simulink model ""  (R2025b)
settings: Solver=ode4  StartTime=0.0  StopTime=300  FixedStep=0.1  RelTol=1e-3
InitFcn:
  | initialization_2d
values from neighbouring files (symbols this model uses):
  d2r = 0.0174532925199    [DDPG_HybridFlocking_agents8-4-1.mat]    (also in flocking_learning.m; initialization_2d.m)
  g = spec(2)    [ActualOutput.m]    (also in DDPG_HybridFlocking_agents8-4-1.mat = 9.806; ModelSwarm.m; initialization.m = 9.806; initialization_2d.m = 9.806)
  m = spec(1)    [ActualOutput.m]    (also in DDPG_HybridFlocking_agents8-4-1.mat = 5; ModelSwarm.m; initialization.m = 15; initialization_2d.m = 5)
  state0 = [435.012620465 721.15936685 20 2.59881408791 0 187.945467124 786.05177403 20 2.90689824266 0 842.493878094 376.880931214 ... (25 elements, 5x5)]    [DDPG_HybridFlocking_agents8-4-1.mat]    (also in flocking_learning.m = zeros(5, N); initialization.m = [x0; y0; z0; V0; gam0; psi0]; initialization_2d.m = [x0; y0; V0; psi0; bank0])
libraries: simulink_extras x10, rllib x6
(part 1 of 2)
settings Model: Creator=chang  LastModifiedBy=laaa

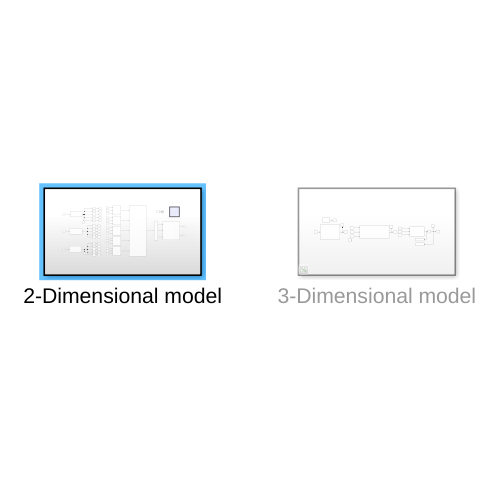
[thumbnail: Simulink's stored preview of the top-level diagram]
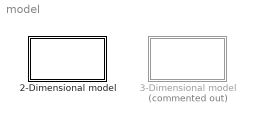
== system model ==
  2-Dimensional model : Subsystem
  3-Dimensional model : Subsystem  Commented=on

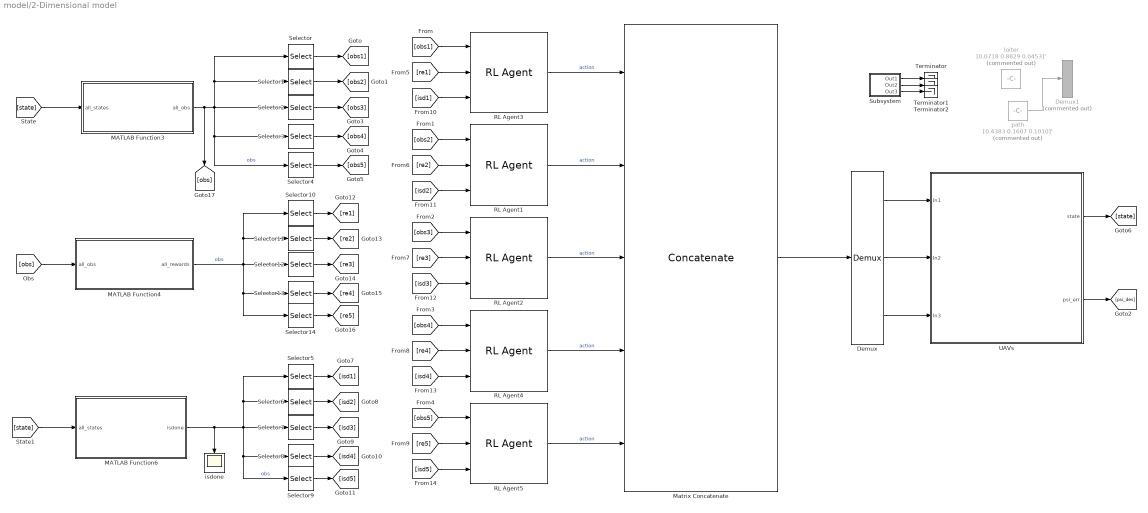
== system model/2-Dimensional model ==
  Demux : Demux  Outputs=3
  Demux1 : Demux  Commented=on  Outputs=3
  MATLAB Function3 : MATLAB Function  TreatAsAtomicUnit=on
  MATLAB Function4 : MATLAB Function  TreatAsAtomicUnit=on
  MATLAB Function6 : MATLAB Function  TreatAsAtomicUnit=on
  Matrix Concatenate : Concatenate  NumInputs=5  Mode=Multidimensional array  ConcatenateDimension=2
  RL Agent{1..5} (5 alike) : rllib/RL Agent  Agent=agent  ExternalActionAsInput=off  ProvideLastAction=off  ProvideCumRwd=off  TreatAsDirectFeedthrough=on  UseStrictObservationDataTypes=off
  Selector : Selector  NumberOfDimensions=2  InputPortWidth=3  IndexOptions=Index vector (dialog),Index vector (dialog)  Indices=1:6,1  OutputSizes=1,1
  Selector1 : Selector  NumberOfDimensions=2  InputPortWidth=3  IndexOptions=Index vector (dialog),Index vector (dialog)  Indices=1:6,2  OutputSizes=1,1
  Selector10 : Selector  NumberOfDimensions=2  InputPortWidth=3  IndexOptions=Index vector (dialog),Index vector (dialog)  Indices=1,1  OutputSizes=1,1
  Selector11 : Selector  NumberOfDimensions=2  InputPortWidth=3  IndexOptions=Index vector (dialog),Index vector (dialog)  Indices=1,2  OutputSizes=1,1
  Selector12 : Selector  NumberOfDimensions=2  InputPortWidth=3  IndexOptions=Index vector (dialog),Index vector (dialog)  Indices=1,3  OutputSizes=1,1
  Selector13 : Selector  NumberOfDimensions=2  InputPortWidth=3  IndexOptions=Index vector (dialog),Index vector (dialog)  Indices=1,4  OutputSizes=1,1
  Selector14 : Selector  NumberOfDimensions=2  InputPortWidth=3  IndexOptions=Index vector (dialog),Index vector (dialog)  Indices=1,5  OutputSizes=1,1
  Selector2 : Selector  NumberOfDimensions=2  InputPortWidth=3  IndexOptions=Index vector (dialog),Index vector (dialog)  Indices=1:6,3  OutputSizes=1,1
  Selector3 : Selector  NumberOfDimensions=2  InputPortWidth=3  IndexOptions=Index vector (dialog),Index vector (dialog)  Indices=1:6,4  OutputSizes=1,1
  Selector4 : Selector  NumberOfDimensions=2  InputPortWidth=3  IndexOptions=Index vector (dialog),Index vector (dialog)  Indices=1:6,5  OutputSizes=1,1
  Selector5 : Selector  NumberOfDimensions=2  InputPortWidth=3  IndexOptions=Index vector (dialog),Index vector (dialog)  Indices=1,1  OutputSizes=1,1
  Selector6 : Selector  NumberOfDimensions=2  InputPortWidth=3  IndexOptions=Index vector (dialog),Index vector (dialog)  Indices=1,2  OutputSizes=1,1
  Selector7 : Selector  NumberOfDimensions=2  InputPortWidth=3  IndexOptions=Index vector (dialog),Index vector (dialog)  Indices=1,3  OutputSizes=1,1
  Selector8 : Selector  NumberOfDimensions=2  InputPortWidth=3  IndexOptions=Index vector (dialog),Index vector (dialog)  Indices=1,4  OutputSizes=1,1
  Selector9 : Selector  NumberOfDimensions=2  InputPortWidth=3  IndexOptions=Index vector (dialog),Index vector (dialog)  Indices=1,5  OutputSizes=1,1
  Subsystem : Subsystem
  Terminator : Terminator
  Terminator1 : Terminator
  Terminator2 : Terminator
  UAVs : Subsystem
  isdone : Scope
      settings: TimeSpan=300  ActiveDisplayYMinimum=-1  ActiveDisplayYMaximum=1  DataLoggingVariableName=ScopeData23
  loiter : Constant  Commented=on  Value=[0.0718 0.8829 0.0453]'
  path : Constant  Commented=on  Value=[0.4383 0.1607 0.1010]'
  wires:
  Demux/3 -> UAVs/3(In3)
  [state] -> MATLAB Function3/1(all_states)
  Demux/2 -> UAVs/2(In2)
  UAVs/2(psi_err) -> [psi_des]
  [obs] -> MATLAB Function4/1(all_obs)
  UAVs/1(state) -> [state]
  path/1 -> Demux1/1
  Demux/1 -> UAVs/1(In1)
  MATLAB Function3/1(all_obs) -> Selector2/1, Selector3/1, Selector4/1, Selector/1, Selector1/1, [obs]  "obs"
  Subsystem/1(Out1) -> Terminator/1
  Subsystem/2(Out2) -> Terminator1/1
  Subsystem/3(Out3) -> Terminator2/1
  [state] -> MATLAB Function6/1(all_states)
  MATLAB Function4/1(all_rewards) -> Selector10/1, Selector11/1, Selector12/1, Selector13/1, Selector14/1  "obs"
  Selector1/1 -> [obs2]
  Selector/1 -> [obs1]
  Selector2/1 -> [obs3]
  Selector3/1 -> [obs4]
  Selector14/1 -> [re5]
  Selector13/1 -> [re4]
  Selector12/1 -> [re3]
  Selector11/1 -> [re2]
  Selector10/1 -> [re1]
  Selector4/1 -> [obs5]
  Selector5/1 -> [isd1]
  Selector9/1 -> [isd5]
  Selector8/1 -> [isd4]
  MATLAB Function6/1(isdone) -> Selector5/1, Selector6/1, Selector7/1, Selector8/1, Selector9/1, isdone/1  "obs"
  Selector6/1 -> [isd2]
  Selector7/1 -> [isd3]
  [re1] -> RL Agent3/2
  [isd1] -> RL Agent3/3
  [obs1] -> RL Agent3/1
  [obs2] -> RL Agent1/1
  [re2] -> RL Agent1/2
  [isd2] -> RL Agent1/3
  [obs3] -> RL Agent2/1
  [re3] -> RL Agent2/2
  [isd3] -> RL Agent2/3
  [obs4] -> RL Agent4/1
  [re4] -> RL Agent4/2
  [isd4] -> RL Agent4/3
  [obs5] -> RL Agent5/1
  [re5] -> RL Agent5/2
  [isd5] -> RL Agent5/3
  RL Agent2/1 -> Matrix Concatenate/3  "action"
  RL Agent4/1 -> Matrix Concatenate/4  "action"
  RL Agent1/1 -> Matrix Concatenate/2  "action"
  RL Agent5/1 -> Matrix Concatenate/5  "action"
  RL Agent3/1 -> Matrix Concatenate/1  "action"
  Matrix Concatenate/1 -> Demux/1

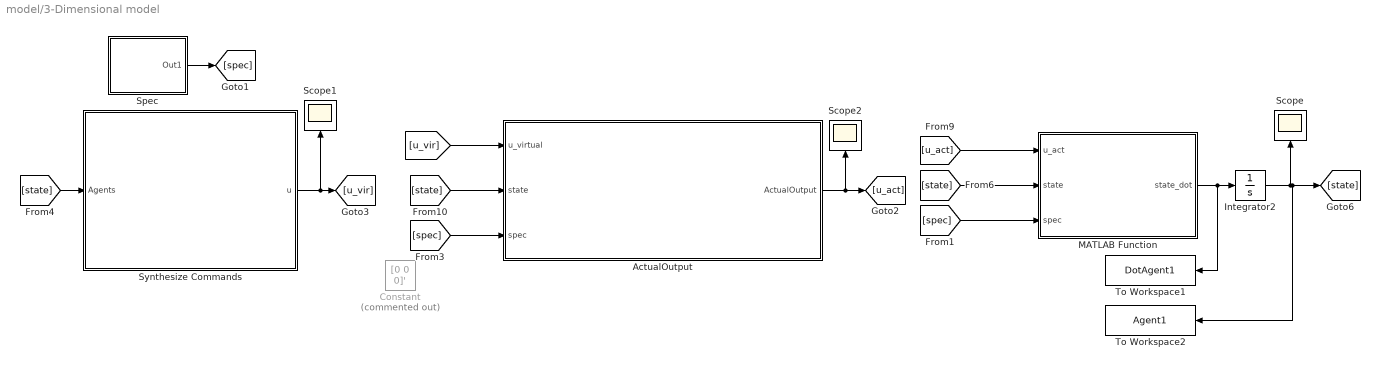
== system model/3-Dimensional model ==
  ActualOutput : Subsystem
  Constant : Constant  Commented=on  Value=[0 0 0]'
  Integrator2 : Integrator  InitialCondition=state0  UpperSaturationLimit=[10^6 ;10^6 ;10^6 ;30 ;15 ;10^6]  LowerSaturationLimit=[-10^6; -10^6 ;-10^6; 0; -15 ;-10^6]'
  MATLAB Function : MATLAB Function  TreatAsAtomicUnit=on
  Scope : Scope
      settings: ActiveDisplayYMinimum=-1796.4442274835574  ActiveDisplayYMaximum=1827.1129411617226
  Scope1 : Scope
      settings: ActiveDisplayYMinimum=-0.625  ActiveDisplayYMaximum=0.625
  Scope2 : Scope
      settings: ActiveDisplayYMinimum=-543.50698903671855  ActiveDisplayYMaximum=2400.6247544411835  DataLoggingVariableName=ScopeData2
  Spec : Subsystem
  Synthesize Commands : Subsystem
  To Workspace1 : ToWorkspace  VariableName=DotAgent1  SaveFormat=Timeseries  SampleTime=-1
  To Workspace2 : ToWorkspace  VariableName=Agent1  SaveFormat=Timeseries  SampleTime=-1
  wires:
  [spec] -> MATLAB Function/3(spec)
  Synthesize Commands/1(u) -> Scope1/1, [u_vir]
  [state] -> ActualOutput/2(state)
  [spec] -> ActualOutput/3(spec)
  [state] -> Synthesize Commands/1(Agents)
  Integrator2/1 -> [state], To Workspace2/1, Scope/1
  [u_vir] -> ActualOutput/1(u_virtual)
  ActualOutput/1(ActualOutput) -> Scope2/1, [u_act]
  MATLAB Function/1(state_dot) -> To Workspace1/1, Integrator2/1
  Spec/1(Out1) -> [spec]
  [state] -> MATLAB Function/2(state)
  [u_act] -> MATLAB Function/1(u_act)

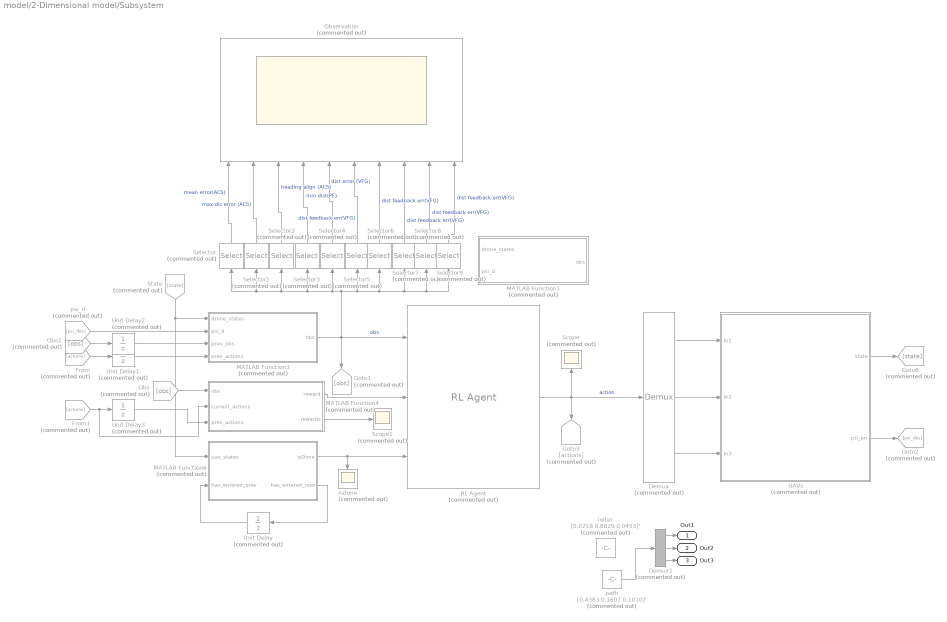
== system model/2-Dimensional model/Subsystem ==
  Demux : Demux  Commented=on  Outputs=3
  Demux1 : Demux  Commented=on  Outputs=3
  From : From  Commented=on  GotoTag=actions
  From1 : From  Commented=on  GotoTag=actions
  Goto1 : Goto  Commented=on  GotoTag=obs
  Goto2 : Goto  Commented=on  GotoTag=psi_des
  Goto3 : Goto  Commented=on  GotoTag=actions
  Goto6 : Goto  Commented=on  GotoTag=state
  MATLAB Function1 : MATLAB Function  Commented=on  TreatAsAtomicUnit=on
  MATLAB Function3 : MATLAB Function  Commented=on  TreatAsAtomicUnit=on
  MATLAB Function4 : MATLAB Function  Commented=on  TreatAsAtomicUnit=on
  MATLAB Function6 : MATLAB Function  Commented=on  TreatAsAtomicUnit=on
  Obs : From  Commented=on  GotoTag=obs
  Obs1 : From  Commented=on  GotoTag=obs
  Observation : Scope  Commented=on  NumInputPorts=10
      settings: TimeSpan=300  TimeDisplayOffset=1  ActiveDisplayYMinimum=0.24464995382973423  ActiveDisplayYMaximum=1.0839277829078073  DataLoggingVariableName=ScopeData20
  RL Agent : rllib/RL Agent  Commented=on  Agent=agent  ExternalActionAsInput=off  ProvideLastAction=off  ProvideCumRwd=off  TreatAsDirectFeedthrough=on  UseStrictObservationDataTypes=off
  Scope : Scope  Commented=on
      settings: TimeSpan=300  ActiveDisplayYMinimum=0.99966044723987579  ActiveDisplayYMaximum=1.0000375956296921  DataLoggingVariableName=ScopeData15
  Scope1 : Scope  Commented=on
      settings: TimeSpan=300  ActiveDisplayYMinimum=-10.882528944657471  ActiveDisplayYMaximum=4.416291277713289  DataLoggingVariableName=ScopeData17
  Selector : Selector  Commented=on  NumberOfDimensions=2  InputPortWidth=3  IndexOptions=Index vector (dialog),Index vector (dialog)  Indices=1,1  OutputSizes=1,1
  Selector1 : Selector  Commented=on  NumberOfDimensions=2  InputPortWidth=3  IndexOptions=Index vector (dialog),Index vector (dialog)  Indices=2,1  OutputSizes=1,1
  Selector2 : Selector  Commented=on  NumberOfDimensions=2  InputPortWidth=3  IndexOptions=Index vector (dialog),Index vector (dialog)  Indices=3,1  OutputSizes=1,1
  Selector3 : Selector  Commented=on  NumberOfDimensions=2  InputPortWidth=3  IndexOptions=Index vector (dialog),Index vector (dialog)  Indices=4,1  OutputSizes=1,1
  Selector4 : Selector  Commented=on  NumberOfDimensions=2  InputPortWidth=3  IndexOptions=Index vector (dialog),Index vector (dialog)  Indices=5,1  OutputSizes=1,1
  Selector5 : Selector  Commented=on  NumberOfDimensions=2  InputPortWidth=3  IndexOptions=Index vector (dialog),Index vector (dialog)  Indices=6,1  OutputSizes=1,1
  Selector6 : Selector  Commented=on  NumberOfDimensions=2  InputPortWidth=3  IndexOptions=Index vector (dialog),Index vector (dialog)  Indices=7,1  OutputSizes=1,1
  Selector7 : Selector  Commented=on  NumberOfDimensions=2  InputPortWidth=3  IndexOptions=Index vector (dialog),Index vector (dialog)  Indices=8,1  OutputSizes=1,1
  Selector8 : Selector  Commented=on  NumberOfDimensions=2  InputPortWidth=3  IndexOptions=Index vector (dialog),Index vector (dialog)  Indices=9,1  OutputSizes=1,1
  Selector9 : Selector  Commented=on  NumberOfDimensions=2  InputPortWidth=3  IndexOptions=Index vector (dialog),Index vector (dialog)  Indices=10,1  OutputSizes=1,1
  State : From  Commented=on  GotoTag=state
  UAVs : Subsystem  Commented=on
  Unit Delay{,1..3} (4 alike) : UnitDelay  Commented=on  SampleTime=-1  HasFrameUpgradeWarning=on
  isdone : Scope  Commented=on
      settings: TimeSpan=300  ActiveDisplayYMinimum=-1  ActiveDisplayYMaximum=1  DataLoggingVariableName=ScopeData12
  loiter : Constant  Commented=on  Value=[0.0718 0.8829 0.0453]'
  path : Constant  Commented=on  Value=[0.4383 0.1607 0.1010]'
  psi_d : From  Commented=on  GotoTag=psi_des
  Out1 : Outport
  Out2 : Outport  Port=2
  Out3 : Outport  Port=3
  wires:
  Unit Delay1/1 -> MATLAB Function3/4(prev_actions)
  Demux/3 -> UAVs/3(In3)
  Obs1/1 -> Unit Delay2/1
  MATLAB Function4/1(reward) -> RL Agent/2
  Selector/1 -> Observation/1  "mean error(ACS)"
  Demux/1 -> UAVs/1(In1)
  From1/1 -> MATLAB Function4/2(current_actions), Unit Delay3/1
  Selector6/1 -> Observation/7  "dist feedback err(VFG)"
  MATLAB Function6/2(has_entered_now) -> Unit Delay/1
  Selector2/1 -> Observation/3  "heading align (ACS)"
  State/1 -> MATLAB Function6/1(uav_states), MATLAB Function3/1(drone_states)
  Selector9/1 -> Observation/10  "dist feedback err(VFG)"
  RL Agent/1 -> Goto3/1, Scope/1, Demux/1  "action"
  Selector1/1 -> Observation/2  "max dis error (ACS)"
  MATLAB Function6/1(isDone) -> RL Agent/3, isdone/1
  From/1 -> Unit Delay1/1
  UAVs/1(state) -> Goto6/1
  Unit Delay2/1 -> MATLAB Function3/3(prev_obs)
  Selector7/1 -> Observation/8  "dist feedback err(VFG)"
  Demux1/2 -> Out2/1
  path/1 -> Demux1/1
  Selector3/1 -> Observation/4  "min dist(PF)"
  MATLAB Function3/1(obs) -> RL Agent/1, Goto1/1, Selector9/1, Selector8/1, Selector7/1, Selector6/1, Selector5/1, Selector/1, Selector1/1, Selector2/1, Selector3/1, Selector4/1  "obs"
  Demux1/1 -> Out1/1
  Demux/2 -> UAVs/2(In2)
  MATLAB Function4/2(rewards) -> Scope1/1
  psi_d/1 -> MATLAB Function3/2(psi_d)
  Unit Delay3/1 -> MATLAB Function4/3(prev_actions)
  UAVs/2(psi_err) -> Goto2/1
  Demux1/3 -> Out3/1
  Unit Delay/1 -> MATLAB Function6/2(has_entered_prev)
  Selector5/1 -> Observation/6  "dist feedback err(VFG)"
  Selector8/1 -> Observation/9  "dist feedback err(VFG)"
  Obs/1 -> MATLAB Function4/1(obs)
  Selector4/1 -> Observation/5  "dist error (VFG)"

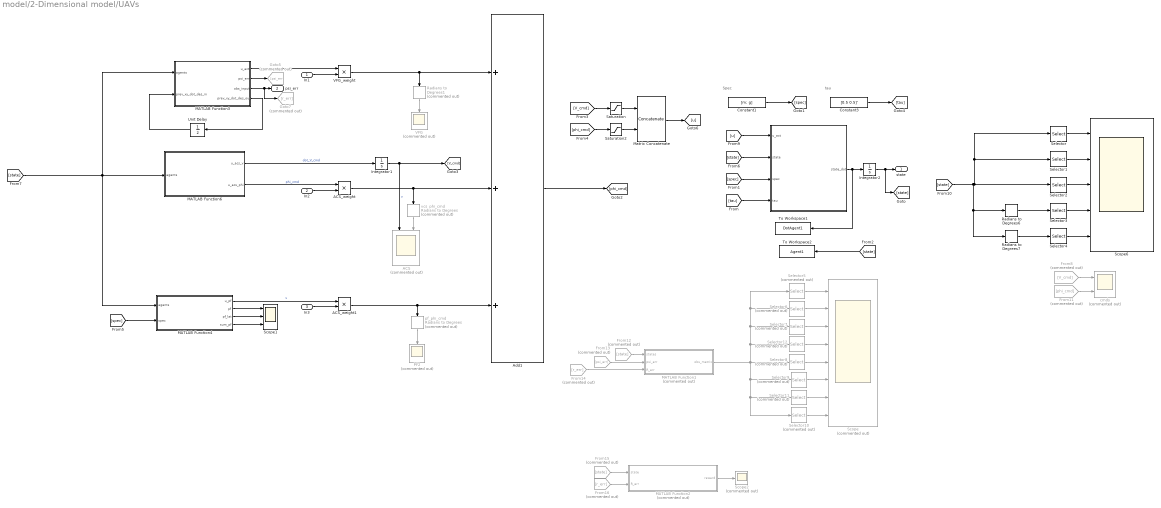
== system model/2-Dimensional model/UAVs ==
  note: Spec
  note: tau
  In1 : Inport
  In2 : Inport  Port=2
  In3 : Inport  Port=3
  " " : MATLAB Function  TreatAsAtomicUnit=on
  ACS : Scope  Commented=on  NumInputPorts=2
      settings: ActiveDisplayYMinimum=-23.869601726691815  ActiveDisplayYMaximum=64.370407175335345  DataLoggingVariableName=ScopeData9
  ACS_weight : Product
  ACS_weight1 : Product
  Add1 : Sum  Inputs=+++
  Constant1 : Constant  Value=[m; g]
  Constant3 : Constant  Value=[0.5 0.5]'
  From11 : From  Commented=on  GotoTag=phi_cmd
  From12 : From  Commented=on  GotoTag=state
  From13 : From  Commented=on  GotoTag=psi_err
  From14 : From  Commented=on  GotoTag=r_err
  From15 : From  Commented=on  GotoTag=state
  From16 : From  Commented=on  GotoTag=r_err
  From8 : From  Commented=on  GotoTag=V_cmd
  Goto5 : Goto  Commented=on  GotoTag=psi_err
  Goto7 : Goto  Commented=on  GotoTag=r_err
  Integrator1 : Integrator  LimitOutput=on  UpperSaturationLimit=35*ones(1,10)  LowerSaturationLimit=15*ones(1,10)
  Integrator2 : Integrator  InitialCondition=state0  LimitOutput=on  UpperSaturationLimit=[10^6; 10^6; 35; 10^6; 30*d2r ]*ones(1,10)  LowerSaturationLimit=[-10^6; -10^6; 15; -10^6; -30*d2r ]*ones(1,10)
  MATLAB Function1 : MATLAB Function  Commented=on  TreatAsAtomicUnit=on
  MATLAB Function2 : MATLAB Function  Commented=on  TreatAsAtomicUnit=on
  MATLAB Function3 : MATLAB Function  TreatAsAtomicUnit=on
  MATLAB Function4 : MATLAB Function  TreatAsAtomicUnit=on
  MATLAB Function6 : MATLAB Function  TreatAsAtomicUnit=on
  Matrix Concatenate : Concatenate  Mode=Multidimensional array
  PF2 : Scope  Commented=on
      settings: TimeSpan=300  ActiveDisplayYMinimum=-44.741397355611163  ActiveDisplayYMaximum=44.744942341518566  DataLoggingVariableName=ScopeData10
  Radians to Degrees1 : simulink_extras/Transformations/Radians to Degrees  Commented=on
  Radians to Degrees6 : simulink_extras/Transformations/Radians to Degrees
  Radians to Degrees7 : simulink_extras/Transformations/Radians to Degrees
  Saturation : Saturate  UpperLimit=35*ones(1,10)  LowerLimit=15*ones(1,10)
  Saturation2 : Saturate  UpperLimit=30*d2r*ones(1,10)  LowerLimit=-30*d2r*ones(1,10)  LinearizeAsGain=off
  Scope : Scope  Commented=on  NumInputPorts=8
      settings: ActiveDisplayString=4  ActiveDisplayYMinimum=0.29571525373676022  ActiveDisplayYMaximum=1.0782538606959156  DataLoggingVariableName=ScopeData18
  Scope1 : Scope  NumInputPorts=3
      settings: ActiveDisplayYMinimum=-1  ActiveDisplayYMaximum=1  DataLoggingVariableName=ScopeData16
  Scope2 : Scope  Commented=on
      settings: ActiveDisplayYMinimum=-109.38583360755611  ActiveDisplayYMaximum=7.8590338705691378  DataLoggingVariableName=ScopeData19
  Scope6 : Scope  NumInputPorts=5
      settings: TimeSpan=300  ActiveDisplayString=5  ShowGrid=off  ActiveDisplayYMinimum=-37.354494394302066  ActiveDisplayYMaximum=37.435243344907619  YLabel=Bank angle (deg)  DataLoggingVariableName=ScopeData13
  Selector : Selector  NumberOfDimensions=2  InputPortWidth=3  IndexOptions=Index vector (dialog),Index vector (dialog)  Indices=1,1:10  OutputSizes=1,1
  Selector1 : Selector  NumberOfDimensions=2  InputPortWidth=3  IndexOptions=Index vector (dialog),Index vector (dialog)  Indices=2,1:10  OutputSizes=1,1
  Selector10 : Selector  Commented=on  NumberOfDimensions=2  InputPortWidth=3  IndexOptions=Index vector (dialog),Index vector (dialog)  Indices=8,1:5  OutputSizes=1,1
  Selector11 : Selector  Commented=on  NumberOfDimensions=2  InputPortWidth=3  IndexOptions=Index vector (dialog),Index vector (dialog)  Indices=7,1:5  OutputSizes=1,1
  Selector12 : Selector  Commented=on  NumberOfDimensions=2  InputPortWidth=3  IndexOptions=Index vector (dialog),Index vector (dialog)  Indices=4,1:5  OutputSizes=1,1
  Selector2 : Selector  NumberOfDimensions=2  InputPortWidth=3  IndexOptions=Index vector (dialog),Index vector (dialog)  Indices=3,1:10  OutputSizes=1,1
  Selector3 : Selector  NumberOfDimensions=2  InputPortWidth=3  IndexOptions=Index vector (dialog),Index vector (dialog)  Indices=4,1:10  OutputSizes=1,1
  Selector4 : Selector  NumberOfDimensions=2  InputPortWidth=3  IndexOptions=Index vector (dialog),Index vector (dialog)  Indices=5,1:10  OutputSizes=1,1
  Selector5 : Selector  Commented=on  NumberOfDimensions=2  InputPortWidth=3  IndexOptions=Index vector (dialog),Index vector (dialog)  Indices=1,1:5  OutputSizes=1,1
  Selector6 : Selector  Commented=on  NumberOfDimensions=2  InputPortWidth=3  IndexOptions=Index vector (dialog),Index vector (dialog)  Indices=2,1:5  OutputSizes=1,1
  Selector7 : Selector  Commented=on  NumberOfDimensions=2  InputPortWidth=3  IndexOptions=Index vector (dialog),Index vector (dialog)  Indices=3,1:5  OutputSizes=1,1
  Selector8 : Selector  Commented=on  NumberOfDimensions=2  InputPortWidth=3  IndexOptions=Index vector (dialog),Index vector (dialog)  Indices=5,1:5  OutputSizes=1,1
  Selector9 : Selector  Commented=on  NumberOfDimensions=2  InputPortWidth=3  IndexOptions=Index vector (dialog),Index vector (dialog)  Indices=6,1:5  OutputSizes=1,1
  To Workspace1 : ToWorkspace  VariableName=DotAgent1  SaveFormat=Timeseries  SampleTime=-1
  To Workspace2 : ToWorkspace  VariableName=Agent1  SaveFormat=Timeseries  SampleTime=-1
  Unit Delay : UnitDelay  SampleTime=-1  HasFrameUpgradeWarning=on
  VFG : Scope  Commented=on
      settings: ActiveDisplayYMinimum=-2.2311275771009429  ActiveDisplayYMaximum=1.6680942354459041  DataLoggingVariableName=ScopeData8
  VFG_weight : Product
  cmds : Scope  Commented=on  NumInputPorts=2
      settings: ActiveDisplayYMinimum=-0.21104649012249277  ActiveDisplayYMaximum=0.44117626715669322  DataLoggingVariableName=ScopeData14
  pf_phi_cmd : simulink_extras/Transformations/Radians to Degrees  Commented=on
  vcs_phi_cmd : simulink_extras/Transformations/Radians to Degrees  Commented=on
  state : Outport
  psi_err : Outport  Port=2
  wires:
  " "/1(state_dot) -> To Workspace1/1, Integrator2/1
  [state] -> MATLAB Function4/1(agents), MATLAB Function3/1(agents), MATLAB Function6/1(agents)
  [spec] -> MATLAB Function4/2(spec)
  MATLAB Function4/1(u_pf) -> ACS_weight1/1  "v"
  MATLAB Function6/2(u_acs_phi) -> ACS_weight/1  "phi_cmd"
  MATLAB Function3/1(u_act) -> VFG_weight/1
  In1/1 -> VFG_weight/2
  VFG_weight/1 -> Radians to Degrees1/1, Add1/1
  Radians to Degrees1/1 -> VFG/1
  MATLAB Function6/1(u_acs_v) -> Integrator1/1  "dot_V_cmd"
  Integrator1/1 -> ACS/1, [V_cmd]  "v"
  ACS_weight/1 -> Add1/2, vcs_phi_cmd/1
  In2/1 -> ACS_weight/2
  vcs_phi_cmd/1 -> ACS/2
  MATLAB Function4/4(sum_pf) -> Scope1/3
  MATLAB Function4/3(pf_lat) -> Scope1/2
  MATLAB Function4/2(pf) -> Scope1/1
  In3/1 -> ACS_weight1/2
  ACS_weight1/1 -> pf_phi_cmd/1, Add1/3
  pf_phi_cmd/1 -> PF2/1
  Add1/1 -> [phi_cmd]
  [V_cmd] -> Saturation/1
  [phi_cmd] -> Saturation2/1
  Saturation/1 -> Matrix Concatenate/1
  Saturation2/1 -> Matrix Concatenate/2
  Matrix Concatenate/1 -> [u]
  [u] -> " "/1(u_act)
  [state] -> " "/2(state)
  [spec] -> " "/3(spec)
  [tau] -> " "/4(tau)
  Constant1/1 -> [spec]
  Constant3/1 -> [tau]
  Integrator2/1 -> [state], state/1
  [state] -> To Workspace2/1
  Selector/1 -> Scope6/1
  Selector1/1 -> Scope6/2
  Selector2/1 -> Scope6/3
  Selector3/1 -> Scope6/4
  Selector4/1 -> Scope6/5
  [state] -> Selector2/1, Selector/1, Selector1/1, Radians to Degrees6/1, Radians to Degrees7/1
  Radians to Degrees6/1 -> Selector3/1
  Radians to Degrees7/1 -> Selector4/1
  From8/1 -> cmds/1
  From11/1 -> cmds/2
  MATLAB Function3/2(psi_err) -> Goto5/1
  MATLAB Function3/3(obs_input) -> Goto7/1, psi_err/1
  From12/1 -> MATLAB Function1/1(states)
  From13/1 -> MATLAB Function1/2(psi_err)
  From14/1 -> MATLAB Function1/3(R_err)
  MATLAB Function1/1(obs_matrix) -> Selector6/1, Selector5/1, Selector7/1, Selector12/1, Selector8/1, Selector9/1, Selector10/1, Selector11/1
  Selector9/1 -> Scope/6
  Selector11/1 -> Scope/7
  Selector10/1 -> Scope/8
  Selector5/1 -> Scope/1
  Selector6/1 -> Scope/2
  Selector7/1 -> Scope/3
  Selector12/1 -> Scope/4
  Selector8/1 -> Scope/5
  From15/1 -> MATLAB Function2/1(state)
  From16/1 -> MATLAB Function2/2(R_err)
  MATLAB Function2/1(reward) -> Scope2/1
  MATLAB Function3/4(prev_xy_dot_des_out) -> Unit Delay/1
  Unit Delay/1 -> MATLAB Function3/2(prev_xy_dot_des_in)

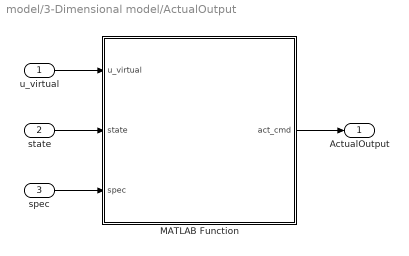
== system model/3-Dimensional model/ActualOutput ==
  u_virtual : Inport
  state : Inport  Port=2
  spec : Inport  Port=3
  MATLAB Function : MATLAB Function  TreatAsAtomicUnit=on
  ActualOutput : Outport
  wires:
  u_virtual/1 -> MATLAB Function/1(u_virtual)
  state/1 -> MATLAB Function/2(state)
  spec/1 -> MATLAB Function/3(spec)
  MATLAB Function/1(act_cmd) -> ActualOutput/1

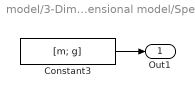
== system model/3-Dimensional model/Spec ==
  Constant3 : Constant  Value=[m; g]
  Out1 : Outport
  wires:
  Constant3/1 -> Out1/1

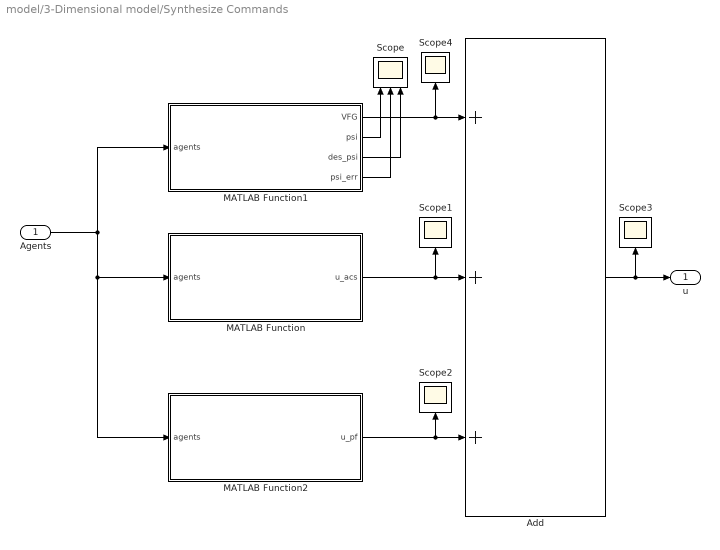
== system model/3-Dimensional model/Synthesize Commands ==
  Agents : Inport
  Add : Sum  Inputs=+++
  MATLAB Function : MATLAB Function  TreatAsAtomicUnit=on
  MATLAB Function1 : MATLAB Function  TreatAsAtomicUnit=on
  MATLAB Function2 : MATLAB Function  TreatAsAtomicUnit=on
  Scope : Scope  NumInputPorts=3
      settings: ActiveDisplayYMinimum=-7.5463075515448264  ActiveDisplayYMaximum=36.500847150660185  DataLoggingVariableName=ScopeData3
  Scope{1..4} (4 alike) : Scope
      Scope1 settings: ActiveDisplayYMinimum=-13.729609129882078  ActiveDisplayYMaximum=15.057455581515576  DataLoggingVariableName=ScopeData4
      Scope2 settings: ActiveDisplayYMinimum=-2.3665763647029392  ActiveDisplayYMaximum=2.4298902475942277  DataLoggingVariableName=ScopeData5
      Scope3 settings: ActiveDisplayYMinimum=-7.2803454393817137  ActiveDisplayYMaximum=5.3802620907689036  DataLoggingVariableName=ScopeData6
      Scope4 settings: ActiveDisplayYMinimum=-15.035450003897875  ActiveDisplayYMaximum=9.9786981173949183  DataLoggingVariableName=ScopeData7
  u : Outport
  wires:
  Agents/1 -> MATLAB Function2/1(agents), MATLAB Function/1(agents), MATLAB Function1/1(agents)
  MATLAB Function1/2(psi) -> Scope/1
  MATLAB Function1/3(des_psi) -> Scope/3
  MATLAB Function1/4(psi_err) -> Scope/2
  MATLAB Function1/1(VFG) -> Add/1, Scope4/1
  MATLAB Function/1(u_acs) -> Scope1/1, Add/2
  MATLAB Function2/1(u_pf) -> Add/3, Scope2/1
  Add/1 -> Scope3/1, u/1

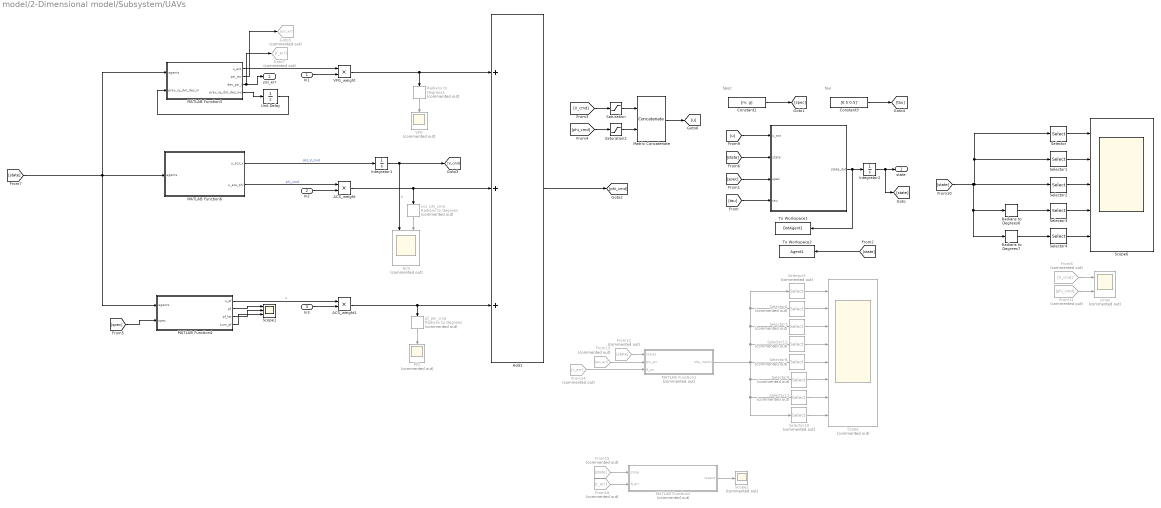
== system model/2-Dimensional model/Subsystem/UAVs ==
  note: Spec
  note: tau
  In1 : Inport
  In2 : Inport  Port=2
  In3 : Inport  Port=3
  " " : MATLAB Function  TreatAsAtomicUnit=on
  ACS : Scope  Commented=on  NumInputPorts=2
      settings: ActiveDisplayYMinimum=-23.869601726691815  ActiveDisplayYMaximum=64.370407175335345  DataLoggingVariableName=ScopeData9
  ACS_weight : Product
  ACS_weight1 : Product
  Add1 : Sum  Inputs=+++
  Constant1 : Constant  Value=[m; g]
  Constant3 : Constant  Value=[0.5 0.5]'
  From11 : From  Commented=on  GotoTag=phi_cmd
  From12 : From  Commented=on  GotoTag=state
  From13 : From  Commented=on  GotoTag=psi_err
  From14 : From  Commented=on  GotoTag=r_err
  From15 : From  Commented=on  GotoTag=state
  From16 : From  Commented=on  GotoTag=r_err
  From8 : From  Commented=on  GotoTag=V_cmd
  Goto5 : Goto  Commented=on  GotoTag=psi_err
  Goto7 : Goto  Commented=on  GotoTag=r_err
  Integrator1 : Integrator  LimitOutput=on  UpperSaturationLimit=35*ones(1,10)  LowerSaturationLimit=15*ones(1,10)
  Integrator2 : Integrator  InitialCondition=state0  LimitOutput=on  UpperSaturationLimit=[10^6; 10^6; 35; 10^6; 30*d2r ]*ones(1,10)  LowerSaturationLimit=[-10^6; -10^6; 15; -10^6; -30*d2r ]*ones(1,10)
  MATLAB Function1 : MATLAB Function  Commented=on  TreatAsAtomicUnit=on
  MATLAB Function2 : MATLAB Function  Commented=on  TreatAsAtomicUnit=on
  MATLAB Function3 : MATLAB Function  TreatAsAtomicUnit=on
  MATLAB Function4 : MATLAB Function  TreatAsAtomicUnit=on
  MATLAB Function6 : MATLAB Function  TreatAsAtomicUnit=on
  Matrix Concatenate : Concatenate  Mode=Multidimensional array
  PF2 : Scope  Commented=on
      settings: TimeSpan=300  ActiveDisplayYMinimum=-44.741397355611163  ActiveDisplayYMaximum=44.744942341518566  DataLoggingVariableName=ScopeData10
  Radians to Degrees1 : simulink_extras/Transformations/Radians to Degrees  Commented=on
  Radians to Degrees6 : simulink_extras/Transformations/Radians to Degrees
  Radians to Degrees7 : simulink_extras/Transformations/Radians to Degrees
  Saturation : Saturate  UpperLimit=35*ones(1,10)  LowerLimit=15*ones(1,10)
  Saturation2 : Saturate  UpperLimit=30*d2r*ones(1,10)  LowerLimit=-30*d2r*ones(1,10)  LinearizeAsGain=off
  Scope : Scope  Commented=on  NumInputPorts=8
      settings: ActiveDisplayString=4  ActiveDisplayYMinimum=0.29571525373676022  ActiveDisplayYMaximum=1.0782538606959156  DataLoggingVariableName=ScopeData18
  Scope1 : Scope  NumInputPorts=3
      settings: ActiveDisplayYMinimum=-1  ActiveDisplayYMaximum=1  DataLoggingVariableName=ScopeData16
  Scope2 : Scope  Commented=on
      settings: ActiveDisplayYMinimum=-109.38583360755611  ActiveDisplayYMaximum=7.8590338705691378  DataLoggingVariableName=ScopeData19
  Scope6 : Scope  NumInputPorts=5
      settings: TimeSpan=300  ActiveDisplayString=5  ShowGrid=off  ActiveDisplayYMinimum=-37.354494394302066  ActiveDisplayYMaximum=37.435243344907619  YLabel=Bank angle (deg)  DataLoggingVariableName=ScopeData13
  Selector : Selector  NumberOfDimensions=2  InputPortWidth=3  IndexOptions=Index vector (dialog),Index vector (dialog)  Indices=1,1:10  OutputSizes=1,1
  Selector1 : Selector  NumberOfDimensions=2  InputPortWidth=3  IndexOptions=Index vector (dialog),Index vector (dialog)  Indices=2,1:10  OutputSizes=1,1
  Selector10 : Selector  Commented=on  NumberOfDimensions=2  InputPortWidth=3  IndexOptions=Index vector (dialog),Index vector (dialog)  Indices=8,1:5  OutputSizes=1,1
  Selector11 : Selector  Commented=on  NumberOfDimensions=2  InputPortWidth=3  IndexOptions=Index vector (dialog),Index vector (dialog)  Indices=7,1:5  OutputSizes=1,1
  Selector12 : Selector  Commented=on  NumberOfDimensions=2  InputPortWidth=3  IndexOptions=Index vector (dialog),Index vector (dialog)  Indices=4,1:5  OutputSizes=1,1
  Selector2 : Selector  NumberOfDimensions=2  InputPortWidth=3  IndexOptions=Index vector (dialog),Index vector (dialog)  Indices=3,1:10  OutputSizes=1,1
  Selector3 : Selector  NumberOfDimensions=2  InputPortWidth=3  IndexOptions=Index vector (dialog),Index vector (dialog)  Indices=4,1:10  OutputSizes=1,1
  Selector4 : Selector  NumberOfDimensions=2  InputPortWidth=3  IndexOptions=Index vector (dialog),Index vector (dialog)  Indices=5,1:10  OutputSizes=1,1
  Selector5 : Selector  Commented=on  NumberOfDimensions=2  InputPortWidth=3  IndexOptions=Index vector (dialog),Index vector (dialog)  Indices=1,1:5  OutputSizes=1,1
  Selector6 : Selector  Commented=on  NumberOfDimensions=2  InputPortWidth=3  IndexOptions=Index vector (dialog),Index vector (dialog)  Indices=2,1:5  OutputSizes=1,1
  Selector7 : Selector  Commented=on  NumberOfDimensions=2  InputPortWidth=3  IndexOptions=Index vector (dialog),Index vector (dialog)  Indices=3,1:5  OutputSizes=1,1
  Selector8 : Selector  Commented=on  NumberOfDimensions=2  InputPortWidth=3  IndexOptions=Index vector (dialog),Index vector (dialog)  Indices=5,1:5  OutputSizes=1,1
  Selector9 : Selector  Commented=on  NumberOfDimensions=2  InputPortWidth=3  IndexOptions=Index vector (dialog),Index vector (dialog)  Indices=6,1:5  OutputSizes=1,1
  To Workspace1 : ToWorkspace  VariableName=DotAgent1  SaveFormat=Timeseries  SampleTime=-1
  To Workspace2 : ToWorkspace  VariableName=Agent1  SaveFormat=Timeseries  SampleTime=-1
  Unit Delay : UnitDelay  SampleTime=-1  HasFrameUpgradeWarning=on
  VFG : Scope  Commented=on
      settings: ActiveDisplayYMinimum=-2.2311275771009429  ActiveDisplayYMaximum=1.6680942354459041  DataLoggingVariableName=ScopeData8
  VFG_weight : Product
  cmds : Scope  Commented=on  NumInputPorts=2
      settings: ActiveDisplayYMinimum=-0.21104649012249277  ActiveDisplayYMaximum=0.44117626715669322  DataLoggingVariableName=ScopeData14
  pf_phi_cmd : simulink_extras/Transformations/Radians to Degrees  Commented=on
  vcs_phi_cmd : simulink_extras/Transformations/Radians to Degrees  Commented=on
  state : Outport
  psi_err : Outport  Port=2
  wires:
  " "/1(state_dot) -> To Workspace1/1, Integrator2/1
  [state] -> MATLAB Function4/1(agents), MATLAB Function3/1(agents), MATLAB Function6/1(agents)
  [spec] -> MATLAB Function4/2(spec)
  MATLAB Function4/1(u_pf) -> ACS_weight1/1  "v"
  MATLAB Function6/2(u_acs_phi) -> ACS_weight/1  "phi_cmd"
  MATLAB Function3/1(u_act) -> VFG_weight/1
  In1/1 -> VFG_weight/2
  VFG_weight/1 -> Add1/1, Radians to Degrees1/1
  Radians to Degrees1/1 -> VFG/1
  MATLAB Function6/1(u_acs_v) -> Integrator1/1  "dot_V_cmd"
  Integrator1/1 -> ACS/1, [V_cmd]  "v"
  ACS_weight/1 -> Add1/2, vcs_phi_cmd/1
  In2/1 -> ACS_weight/2
  vcs_phi_cmd/1 -> ACS/2
  MATLAB Function4/4(sum_pf) -> Scope1/3
  MATLAB Function4/3(pf_lat) -> Scope1/2
  MATLAB Function4/2(pf) -> Scope1/1
  In3/1 -> ACS_weight1/2
  ACS_weight1/1 -> pf_phi_cmd/1, Add1/3
  pf_phi_cmd/1 -> PF2/1
  Add1/1 -> [phi_cmd]
  [V_cmd] -> Saturation/1
  [phi_cmd] -> Saturation2/1
  Saturation/1 -> Matrix Concatenate/1
  Saturation2/1 -> Matrix Concatenate/2
  Matrix Concatenate/1 -> [u]
  [u] -> " "/1(u_act)
  [state] -> " "/2(state)
  [spec] -> " "/3(spec)
  [tau] -> " "/4(tau)
  Constant1/1 -> [spec]
  Constant3/1 -> [tau]
  Integrator2/1 -> [state], state/1
  [state] -> To Workspace2/1
  Selector/1 -> Scope6/1
  Selector1/1 -> Scope6/2
  Selector2/1 -> Scope6/3
  Selector3/1 -> Scope6/4
  Selector4/1 -> Scope6/5
  [state] -> Selector2/1, Selector/1, Selector1/1, Radians to Degrees6/1, Radians to Degrees7/1
  Radians to Degrees6/1 -> Selector3/1
  Radians to Degrees7/1 -> Selector4/1
  From8/1 -> cmds/1
  From11/1 -> cmds/2
  MATLAB Function3/2(psi_err) -> Goto5/1
  MATLAB Function3/3(des_psi_i) -> psi_err/1, Goto7/1
  From12/1 -> MATLAB Function1/1(states)
  From13/1 -> MATLAB Function1/2(psi_err)
  From14/1 -> MATLAB Function1/3(R_err)
  MATLAB Function1/1(obs_matrix) -> Selector6/1, Selector5/1, Selector7/1, Selector12/1, Selector8/1, Selector9/1, Selector10/1, Selector11/1
  Selector9/1 -> Scope/6
  Selector11/1 -> Scope/7
  Selector10/1 -> Scope/8
  Selector5/1 -> Scope/1
  Selector6/1 -> Scope/2
  Selector7/1 -> Scope/3
  Selector12/1 -> Scope/4
  Selector8/1 -> Scope/5
  From15/1 -> MATLAB Function2/1(state)
  From16/1 -> MATLAB Function2/2(R_err)
  MATLAB Function2/1(reward) -> Scope2/1
  MATLAB Function3/4(prev_xy_dot_des_out) -> Unit Delay/1
  Unit Delay/1 -> MATLAB Function3/2(prev_xy_dot_des_in)

== matlab function 2-Dimensional model/Subsystem/MATLAB Function3 ==
  data: obs output size=10; drone_states input; psi_d input; prev_obs input; prev_actions input
function obs = get_observation_swarm(drone_states, psi_d, prev_obs, prev_actions)
    %#codegen
    %% --- [설계 파라미터] ---
    R_acs = 50;      % 드론 간 희망 간격
    R_target = 500;  % 목표 원 궤도 반지름
    
    N = size(drone_states, 2);
    pos = drone_states(1:2, :); 
    psi = drone_states(4, :);   
    
    % 1. 군집 중심(Centroid) 및 반지름 계산
    dist_from_center = sqrt(sum(pos.^2, 1));
    mean_radius = mean(dist_from_center); % 군집의 평균 반지름 (중심점 역할)
    std_radius = std(dist_from_center);   % 군집이 얼마나 퍼져있는지 (응집도)

    % 2. 군집 중심의 경로 오차 (Dead-zone 30m 적용)
    % 개별 드론이 아닌 '중심'이 궤도 근처(±30m)에만 있으면 오차를 0으로 간주
    path_err_centroid = mean_radius - R_target;
    if abs(path_err_centroid) < 30
        obs_path = 0.0;
    else
        obs_path = tanh(path_err_centroid / 150); 
    end

    % 3. 간격 오차 (대형 유지 상태)
    dist_matrix = pdist2(pos', pos');
    dist_matrix(logical(eye(N))) = inf;
    d_min_each = min(dist_matrix, [], 2);
    obs_spacing = mean(abs(d_min_each - R_acs)) / R_acs;

    % 4. 헤딩 정렬 (군집 전체의 방향성)
    avg_psi = atan2(mean(sin(psi)), mean(cos(psi)));
    obs_alignment = (1 - cos(psi_d - avg_psi));

    % 5. 변화량 및 피드백 정보
    obs_delta = tanh((obs_path - prev_obs(2)) * 10); % 경로 오차 변화량

    % 최종 10차원 관측 벡터 (시뮬링크 고정 크기 대응)
    obs = zeros(10, 1, 'double');
    obs(1) = min(obs_spacing, 1.0);    % 대형 유지 오차
    obs(2) = obs_path;                % 군집 중심의 궤도 오차
    obs(3) = obs_alignment;           % 헤딩 정렬 오차
    obs(4) = obs_delta;               % 오차 변화량 (Progress 동력)
    obs(5) = min(std_radius / 100, 1.0); % 군집 분산 (퍼짐 정도)
    obs(6) = prev_actions(1);         % 이전 VFG 가중치
    obs(7) = prev_actions(2);         % 이전 ACS 가중치
    obs(8) = prev_actions(3);         % 이전 PF 가중치
    obs(9) = exp(-min(d_min_each)/20); % 최인접 드론 위험도 (PF)
    obs(10) = mean_radius / 1000;     % 전체적인 스케일 정보
end

== matlab function 2-Dimensional model/Subsystem/MATLAB Function6 ==
  data: uav_states input; isDone output; has_entered_prev input; has_entered_now output
function [isDone, has_entered_now] = check_termination(uav_states, has_entered_prev)
    % 입력 파라미터:
    has_entered_now = has_entered_prev;
    isDone = 0; 

    pos_NE = uav_states(1:2, :); % [2 x 20] 행렬 (North, East)
    V_vec = uav_states(3, :);    % [1 x 20] 행렬 (Velocity)
    % dist_to_center = sqrt(sum(pos_NE.^2, 1)); 
    % 
    % max_range_default = 2500.0; % 궤도 진입 전 최대 허용 범위
    % max_range_locked = 700.0;   % 궤도 진입 후 엄격한 제한 범위
    % orbit_radius = 500.0;       % 목표 궤도
    % entry_threshold = 0.0;     % 궤도 근처(500±50m) 진입 판단 기준

    %% 2. 속도 제한 체크 (기존 작성 코드)
    if max(V_vec) > 40
        isDone = 1;
    end    

    %% 4. 작전 구역 이탈 체크 (Geofencing)
    
    % 궤도 진입 판정 (한 대라도 궤도 근처에 도달하면 락온!)
    % if any(abs(dist_to_center - orbit_radius) < entry_threshold)
    %     has_entered_now = 1;
    % end
    
    % 가변 범위 적용
    % if has_entered_now
    %     current_max = max_range_locked; % 궤도 들어온 후엔 700m만 넘어도 끝!
    % else
    %     current_max = max_range_default; % 그 전엔 2500m까지 봐줌
    % end
    
    % 종료 조건 판정
    % if any(dist_to_center > current_max)
    %     isDone = 1;
    %     has_entered_now = 0; % 종료 시 초기화
    % end
    
    %% 5. (선택 사항) 최소 속도 체크 (Stall 방지)
    if min(V_vec) < 10
        isDone = 1;
    end
    %% [추가] 6. 충돌 체크 (가장 중요!)
    % dist_matrix = pdist(pos_NE'); % 드론 간 거리 계산
    % if ~isempty(dist_matrix)
    %     if min(dist_matrix) < 5 % d_crash 기준 (예: 5m)
    %         isDone = 1; % 부딪히면 그 즉시 에피소드 종료!
    %     end
    % end
end

== matlab function 2-Dimensional model/Subsystem/UAVs/MATLAB Function3 ==
  data: u_act output; agents input; psi_err output; des_psi_i output; prev_xy_dot_des_in input; prev_xy_dot_des_out output
function [u_act, psi_err, des_psi_i, prev_xy_dot_des_out]  = VFG(agents,prev_xy_dot_des_in)
    % agents: [x; y; V; psi; theta] (5 x N 행렬)
    
    % --- 설정값 ---
    N = size(agents, 2);
    dt = 0.1;
    xt = 0; yt = 0;   
    Vd = 20;          % 드론이 유지해야 할 목표 속도 (m/s)
    rd = 500;         
    g = 9.806;        
    K_vf = 1.5;  
    psi_err = zeros(1,N);
    r_err = zeros(1,N);
    % curr_xy_dot_des_out = zeros(2, N); % 다음 스텝을 위해 밖으로 내보냄
    prev_xy_dot_des_out = zeros(2, N);
    % 출력 변수 초기화 (u_act: 2 x N)
    u_act = zeros(1, N);
    % des_psi = zeros(1, N);
    % psi_err = zeros(1, N);

    for i = 1 : N
        %% 1. 현재 상태 추출
        x = agents(1,i);
        y = agents(2,i);
        V = agents(3,i);      
        psi = agents(4,i);    
        
        %% 2. Vector Field 계산 (Orbit Guidance)
        xr = x - xt;
        yr = y - yt;
        r = sqrt(xr^2 + yr^2);
        r_safe = max(r, 0.1); 
        
        term1 = r_safe^2 - rd^2;
        term2 = 2 * r_safe * rd;
        
        % Vector Field 방향 생성
        xy_dot_dir = [ (term1 * xr + term2 * yr);
                       (term1 * yr - term2 * xr) ];
        
        % 현재 시점의 목표 속도 벡터
        curr_xy_dot_des = -(Vd / (r_safe * (r_safe^2 + rd^2))) * xy_dot_dir;
        % curr_xy_dot_des = xy_dot_dir;
        
        %% 3. 목표 가속도 생성 (수치 미분)
        xy_ddot_des = (curr_xy_dot_des - prev_xy_dot_des_in(:,i)) / dt;
        
        %% 4. 목표 헤딩율(dot_psi_d) 계산
        % N,E_dot
        dot_N = curr_xy_dot_des(1);
        dot_E = curr_xy_dot_des(2);

        % N,E_ddot
        % r_dot = (xr*dot_N + yr*dot_E)/r_safe;
        % ddot_N = dot_N*(r_safe^2-rd^2) - 2*xr*r_safe*r_dot + 2*rd*(dot_E*r_safe + yr*r_dot);
        % ddot_E = dot_E*(r_safe^2-rd^2) - 2*yr*r_safe*r_dot + 2*rd*(dot_N*r_safe + xr*r_dot);
        ddot_N = xy_ddot_des(1);
        ddot_E = xy_ddot_des(2);

        % desired psi
        des_psi_i = atan2(dot_E, dot_N);
        % atan2(sin, cos) 방식이 오차 계산 시 가장 안전합니다.
        % err = atan2(sin(des_psi_i - psi), cos(des_psi_i - psi));
        psi_wrapped = atan2(sin(psi), cos(psi));
        err = des_psi_i - psi_wrapped;
        % [중요] Reddit 로직: 180도(pi)를 넘어가면 반대 방향 최단거리로 보정
        if err > pi
            err = err - 2*pi;
            elseif err < -pi
                err = err + 2*pi;
        end

        psi_err(i) = err;
        r_err(i) = r;


        % desired psi_dot
        vel_sq_safe = max(dot_N^2 + dot_E^2, 0.01); 
        dot_psi_d = (ddot_E * dot_N - dot_E * ddot_N) / vel_sq_safe;
        
        %% 6. 최종 제어 입력 생성 (u_act: 2 x N)
        % 1행: 속도 명령 (멈춰있으면 안 되므로 Vd 또는 현재 V를 넣어줍니다)

        
        % 2행: 뱅크각(Roll) 명령
        u_act(1, i) = atan2(V*(dot_psi_d + K_vf * err), g);
        
        % 결과 저장
        % des_psi(i) = des_psi_i;
        % psi_err(i) = err;
        
        % 상태 업데이트
        prev_xy_dot_des_out(:,i) = curr_xy_dot_des;
    end
end

== matlab function 2-Dimensional model/Subsystem/UAVs/MATLAB Function4 ==
  data: u_pf output; agents input; spec input; pf output; pf_lat output; sum_pf output
function [u_pf, pf, pf_lat, sum_pf]  = PF(agents, spec)

    %% params
    % idx = 1;
    N = size(agents,2);
    alp = 9; % Potential Strength
    % Bell Function Constant (a, b, c)
    a   = 10; 
    b   = 2;
    c   = 20;
    u_pf = zeros(1,N);
    pf = zeros(1,N);
    denominator = 0;
    sum_pf = zeros(2,N);

    g = spec(2);

    %% Algorithm
    for idx = 1: N
        pos_i = agents(1:2, idx);
        psi = agents(4, idx);
        sum = zeros(2,1);

        for j = 1: N
            if idx==j 
                continue; 
            end
            pos_j = agents(1:2, j);
            pos_ij = pos_i - pos_j;
            pos_ji = pos_j - pos_i;
            norm_ij = norm(pos_ij);
    
            val = (norm_ij - c)/a;
            denominator = 1 + val^(2*b);
            if norm_ij > 0.001
                sum = sum + (alp/denominator)*(pos_ji/norm_ij);
            end
        end
        pf_lat = [-sin(psi) cos(psi)]*[sum(1); sum(2)];
        phi_cmd = atan2(pf_lat, g);
        u_pf(1,idx) = phi_cmd;
        pf(1,idx) = denominator; 
        sum_pf(:,idx) = sum;
    end
end

== matlab function 2-Dimensional model/Subsystem/UAVs/MATLAB Function6 ==
  data: u_acs_v output; agents input; u_acs_phi output
function [u_acs_v, u_acs_phi] = ACS(agents)
    N           = size(agents, 2);
    u_acs_v     = zeros(1, N);
    u_acs_phi   = zeros(1, N);

    % Parameters
    lambda      = 1;  % CS gain
    sigma       = 1;   % ACS gain (논문의 sigma)
    beta        = 0.4;
    R           = 50;        % Desired distance
    K1          = 0.5;     % Damping
    K2          = 0.05;      % Spring
    g           = 9.806;

    if N < 2, return; end

    for i = 1:N
        %% i agent state
        pos_i       = agents(1:2, i);
        V_i         = agents(3, i);
        psi_i       = agents(4, i);
        % vel_Ni,Ei
        vel_i       = [V_i*cos(psi_i); V_i*sin(psi_i)];
        
        % Initiatializaton
        sum_acs_lon = 0;
        sum_acs_lat = 0;
        sum_cs_lon  = 0;
        sum_cs_lat  = 0;

        for j = 1:N

            if i == j, continue; end
            %% j agent state
            pos_j       = agents(1:2, j);
            V_j         = agents(3, j);
            psi_j       = agents(4, j);
            % vel_Nj,Ej
            vel_j       = [V_j*cos(psi_j); V_j*sin(psi_j)];

            rel_pos_ij = pos_i - pos_j; % (x_i - x_j)
            rel_pos_ji = pos_j - pos_i; % (x_j - x_i)
            rel_vel_ij = vel_i - vel_j; % (v_i - v_j)
            rel_vel_ji = vel_j - vel_i; % (v_j - v_i)
            r_ij        = norm(rel_pos_ij); % L2 Norm

            if r_ij < 1e-3, r_ij = 1e-3; end

            % Cucker-Smale Term (Alignment)
            eta_ij  = 1 / ((1 + r_ij^2)^beta); % communication deday rate
            % Augmented Term (Bonding Force)
            bond1   = (K1/(2*r_ij^2)) * dot(rel_vel_ij, rel_pos_ij); % damping
            bond2   = (K2/(2*r_ij)) * (r_ij - 2*R); % spring
            nu_ij   =  bond1 + bond2;

            % londitudinal force
            cs_lon  = eta_ij * (rel_vel_ji(1)*cos(psi_i) + rel_vel_ji(2)*sin(psi_i));
            acs_lon = nu_ij * (rel_pos_ji(1)*cos(psi_i) + rel_pos_ji(2)*sin(psi_i));
            % lateral force
            cs_lat  = eta_ij * (-rel_vel_ji(1)*sin(psi_i) + rel_vel_ji(2)*cos(psi_i));
            acs_lat = nu_ij * (-rel_pos_ji(1)*sin(psi_i) + rel_pos_ji(2)*cos(psi_i));

            % sum
            sum_cs_lon  = sum_cs_lon + cs_lon;
            sum_acs_lon = sum_acs_lon + acs_lon;
            sum_cs_lat  = sum_cs_lat + cs_lat;
            sum_acs_lat = sum_acs_lat + acs_lat;
        end
        % psi_dot_cmd =  (lambda/N)*sum_cs_lat; 
        % u_acs_theta(i) = (lambda/N*g)*sum_cs_lat + (sigma/N) * sum_lat; 

        u_acs_v(i)      = (lambda/N)*sum_cs_lon + (sigma/N)*sum_acs_lon;
        % u_acs_v(i)      = (sigma/N)*sum_acs_lon;
        psi_dot_cmd     = (lambda/N)*sum_cs_lat + (sigma/N)*sum_acs_lat; 
        u_acs_phi(i)    = atan2(psi_dot_cmd, g);
        % u_acs_theta(i) = 0;

    end
end

== matlab function 2-Dimensional model/Subsystem/MATLAB Function1 ==
  data: obs output size=9; drone_states input; psi_d input
function obs = get_observation(drone_states, psi_d)
    % drone_states: 5 x N 행렬 (x, y, z, v, psi, phi)
    % path_info: 현재 군집 중심에서 가장 가까운 경로 점 정보

    obs = zeros(9,1);
    
    % N = 10;
    v = drone_states(3, :);
    psi = drone_states(4, :);
    phi = drone_states(5, :);
    pos = drone_states(1:2, :); % x, y 위치

    % 1. VFG 지표
    center_pos = mean(pos, 2);
    R_orbit = 500;
    dist_from_origin = norm(center_pos); 
    track_error = abs(dist_from_origin - R_orbit);
    
    avg_cos = mean(cos(psi));
    avg_sin = mean(sin(psi));
    avg_psi = atan2(avg_sin, avg_cos);
    
    psi_err = psi_d - avg_psi; % Delta psi
    % obs_vfg = [track_error, sin(psi_err), cos(psi_err)];

    % 2. ACS 지표
    v_std = std(v); % O_v,std
    alignment = sqrt(avg_cos^2 + avg_sin^2); % O_align

    relative_pos = pos - center_pos; 
    all_distances = vecnorm(relative_pos, 2, 1); 

    max_dist_from_center = max(all_distances);
    % obs_acs = [v_std, alignment, max_dist_from_center];

    % 3. PF 지표
    % [PF] - 안전장치 
    dist_matrix = pdist(pos');
    if isempty(dist_matrix)
        min_dist = 1000.0; % 거리가 멀다고 가정 (충돌 방지 페널티 안 받게)
        % energy = 0.0;
    else
        min_dist = min(dist_matrix);
        % energy = 0.0;
        % a = 0.1; d_safe = 75;
        % for i = 1:length(dist_matrix)
        %     if dist_matrix(i) < d_safe
        %         energy = energy + exp(-a * (dist_matrix(i) - d_safe));
        %     end
        % end
    end
    % obs_pf = [min_dist, energy];

    % 4. Self 지표 (평균 상태)
    % obs_self = [mean(v), mean(phi)];

    % 최종 Observation 벡터 (10차원)
    % obs = [obs_vfg, obs_acs, obs_pf, obs_self]';

    s_track_error = min(track_error / 500, 1);      % 거리 오차 
    s_sin_psi     = sin(psi_err);                % 방향 오차
    s_cos_psi     = cos(psi_err);                % 방향 오차
    
    s_v_std       = min(v_std / 20, 1);          % 속도 편차 (10m/s 기준)
    s_alignment   = alignment;                    % 정렬도 (이미 0~1)
    s_max_dist    = min(max_dist_from_center / 300, 1); % 군집 반경
    s_energy_dist = (75 - min_dist) / 75;
    s_energy_dist = max(0, min(s_energy_dist, 1));

    % 최종 관측값: 제곱을 해서 거리가 가까워질수록 벌점이 기하급수적으로 커지게 함
    s_energy_mapped = s_energy_dist^2;
    % s_energy      = tanh(energy / 50);           % PF 에너지 (50단위 포화)
    
    % s_mean_v      = mean(v) / 20;                % 평균 속도 (Max 30 가정)
    % s_mean_phi    = mean(phi) / (30*180/pi);          % 평균 뱅크각 (Max 45도 가정)

    % 최종 10차원 벡터 반환
    obs = [s_track_error; s_sin_psi; s_cos_psi; s_v_std; s_alignment; ...
           s_max_dist; s_energy_mapped;  mean(v); mean(phi)];
end

== matlab function 2-Dimensional model/MATLAB Function3 ==
  data: all_obs output size=10; all_states input
function all_obs = get_observation_normalized(all_states)
    % path_info 대신 내부 상수로 관리 (필요 시 수정)
    num_agents = 5; % 에이전트 수 통일
    obs_dim = 8;
    R_safe = 20;
    R_freedom = 50;
    target_rd = 500;
    
    all_obs = zeros(obs_dim, num_agents);
    all_pos = all_states(1:2, :)'; 
    center_pos = mean(all_pos, 1);
    r_c = norm(center_pos);
    avg_psi = atan2(mean(sin(all_states(4,:))), mean(cos(all_states(4,:))));

    for i = 1:num_agents
        pos_i = all_states(1:2, i)';
        V_i = all_states(3, i);
        psi_i = all_states(4, i);
        gamma_i = all_states(5, i);

        % 정규화 로직
        center_path_err_norm = tanh(abs(r_c - target_rd) / 100); 
        psi_align_err = atan2(sin(psi_i - avg_psi), cos(psi_i - avg_psi));
        norm_psi_align = (psi_align_err / pi + 1) / 2;
        dist_to_center = norm(pos_i - center_pos);
        norm_dist_center = min(max(dist_to_center / R_freedom, 0), 1); 
        
        min_dist = inf;
        for j = 1:num_agents
            if i ~= j
                d_ij = norm(pos_i - all_states(1:2, j)');
                if d_ij < min_dist, min_dist = d_ij; end
            end
        end
        norm_min_dist = min(max(min_dist / R_safe, 0), 1);
        norm_speed = tanh(V_i / 20);
        norm_gamma = (gamma_i / (pi/2) + 1) / 2;

        all_obs(:, i) = [center_path_err_norm; norm_psi_align; norm_dist_center; ...
                         norm_min_dist; norm_speed; norm_gamma];
    end
end

== matlab function 2-Dimensional model/MATLAB Function4 ==
  data: all_obs input; all_rewards output
function all_rewards = get_reward_normalized(all_obs)
    % is_crash_vec를 별도로 받기 번거롭다면 obs(4) 즉 norm_min_dist를 활용하세요
    num_agents = 5;
    all_rewards = zeros(1, num_agents);
    sigma_path = 0.2; sigma_align = 0.3; gamma_col = 0.1;

    for i = 1:num_agents
        obs_i = all_obs(:, i);
        
        F_path = exp(-(obs_i(1)^2) / (2 * sigma_path^2));
        F_align = exp(-((obs_i(2)-0.5)*2)^2 / (2 * sigma_align^2));
        
        if obs_i(3) < 0.8
            F_freedom = 1.0; 
        else
            F_freedom = exp(-( (obs_i(3) - 0.8)^2 ) / 0.1);
        end
        
        % 충돌 회피 (obs_i(4)가 0에 가까워지면 보상이 급격히 하락)
        F_col = (obs_i(4)^2) / ( (1 - obs_i(4) + gamma_col)^2 );
        F_col = min(F_col, 1);
        
        F_spd = obs_i(5);

        % 곱셈형 보상 산출
        all_rewards(i) = F_path * F_align * F_freedom * F_col * F_spd;
        
        % [추가] 강제 페널티: 안전거리가 20% 미만(2m)이면 보상을 0으로
        if obs_i(4) < 0.2
            all_rewards(i) = 0;
        end
    end
end

== matlab function 2-Dimensional model/MATLAB Function6 ==
  data: all_states input; isdone output
function isdone = check_termination(all_states)
    isdone = false;
    center_pos = mean(all_states(1:2, :), 2);
    r_c = norm(center_pos);
    
    % 1. 궤도 이탈 (너무 멀어지거나 가까워지면 종료)
    if r_c < 250 || r_c > 750
        isdone = true;
        return;
    end
    
    % 2. 고도나 속도 등 물리적 한계 초과 시 종료 로직 추가 가능
    if any(all_states(3,:) < 5) % 속도가 너무 느려져도 추락으로 간주
        isdone = true;
        return;
    end
end
